simulink model "UrbanCHIL"  (Simulink 8.1)
settings: Solver=ode1  StartTime=0.0  StopTime=inf  FixedStep=Ts  MaxStep=1e-3  RelTol=1e-3
PostLoadFcn:
  | NREL_Mode=1; BANSHEE_init;
InitFcn:
  | NREL_Mode=1; BANSHEE_init;
values from neighbouring files (symbols this model uses):
  DER_REL = xlsread('DER_relay.xlsx')    [relay_settings_init.m]
  F0 = xlsread('F0_relay_banshee.xlsx')    [relay_settings_init.m]
  F2 = xlsread('F2_relay_banshee.xlsx')    [relay_settings_init.m]
  F3 = xlsread('F3_relay_banshee.xlsx')    [relay_settings_init.m]
  F4 = xlsread('F4_relay_nrel.xlsx')    [relay_settings_init.m]
  Ts = 100E-6    (= 0.0001)    [BANSHEE_init.m]    (also in Ghost_init.m)
undefined symbols (not defined in the file or in its folder): CBID, communications_lib, Feeder2_lib, Feeder3_lib, Feeder4_lib, generic_ethernet_cb, Left, relay_housing_lib, SM_UtilityService, SS_COMMUNICATION, SS_F2_RELAY_HOUSING, SS_F3_RELAY_HOUSING, SS_Feeder2, SS_Feeder3, SS_Feeder4, Stim, type, utility_service_lib, V
libraries: simulink x80, relay_modbus_lib x80, breaker_lib x46, rtio_generic_modbus x45, cables_lib x30, rtlab x22, Load_lib x21, powerlib x20, transformer_lib x19, ssn_lib x13, artemis x6, BESS_lib x4
(part 4 of 6)

== system UrbanCHIL/SC_ctrl/PV2 control ==
  note: Use Modbus from
      | Console
  note: Use Modbus TCP
  Bus Creator1 : BusCreator  Inputs=3
  Bus Creator12 : BusCreator  Inputs=8
  Gain3 : Gain  Gain=1000
  Gain4 : Gain  Gain=1000
  Gain5 : Gain  Gain=4800
  Gain6 : Gain  Gain=6000
  Manual Switch : ManualSwitch  CurrentSetting=0
  Manual Switch1 : ManualSwitch  CurrentSetting=0
  Manual Switch2 : ManualSwitch
  Manual Switch3 : ManualSwitch  CurrentSetting=0
  PCmd{1..2,4,6} (4 alike) : Constant  Value=0
  PCmd3 : Constant
  PCmd5 : Constant  Value=11
  PCmd7 : Constant
  PCmd8 : Constant
  Rate Transition : RateTransition  Deterministic=off
  S Profile1 : simulink/Sources/Repeating Sequence Stair  OutValues=Stim.PV2.Ena  tsamp=[Stim.Ts Ts]  OutMin=[]  OutMax=[]  OutDataTypeStr=Inherit: Inherit via back propagation  OutDataType=fixdt(0,8)  ConRadixGroup=Best Precision: Vector-wise  OutScaling=2^-12
  S Profile2 : simulink/Sources/Repeating Sequence Stair  OutValues=Stim.ESS2.p  tsamp=[Stim.Ts Ts]  OutMin=[]  OutMax=[]  OutDataTypeStr=Inherit: Inherit via back propagation  OutDataType=fixdt(0,8)  ConRadixGroup=Best Precision: Vector-wise  OutScaling=2^-12
  S Profile3 : simulink/Sources/Repeating Sequence Stair  OutValues=Stim.ESS2.q  tsamp=[Stim.Ts Ts]  OutMin=[]  OutMax=[]  OutDataTypeStr=Inherit: Inherit via back propagation  OutDataType=fixdt(0,8)  ConRadixGroup=Best Precision: Vector-wise  OutScaling=2^-12
  S Profile4 : simulink/Sources/Repeating Sequence Stair  OutValues=Stim.ESS2.v  tsamp=[Stim.Ts Ts]  OutMin=[]  OutMax=[]  OutDataTypeStr=Inherit: Inherit via back propagation  OutDataType=fixdt(0,8)  ConRadixGroup=Best Precision: Vector-wise  OutScaling=2^-12
  S Profile5 : simulink/Sources/Repeating Sequence Stair  OutValues=Stim.ESS2.f  tsamp=[Stim.Ts Ts]  OutMin=[]  OutMax=[]  OutDataTypeStr=Inherit: Inherit via back propagation  OutDataType=fixdt(0,8)  ConRadixGroup=Best Precision: Vector-wise  OutScaling=2^-12
  Tuning : Subsystem
  Out1 : Outport
  wires:
  Manual Switch3/1 -> Bus Creator12/1  "Ctrl"
  PCmd8/1 -> Manual Switch3/2
  S Profile5/1 -> Gain6/1
  Manual Switch/1 -> Gain3/1
  Bus Creator12/1 -> Bus Creator1/1  "ModbusFromSC"
  Manual Switch1/1 -> Gain4/1
  S Profile4/1 -> Gain5/1
  PCmd4/1 -> Manual Switch1/2
  PCmd3/1 -> Manual Switch/2
  S Profile2/1 -> Manual Switch/1
  S Profile3/1 -> Manual Switch1/1
  S Profile1/1 -> Manual Switch3/1
  PCmd1/1 -> Bus Creator12/6
  PCmd2/1 -> Bus Creator12/7
  PCmd5/1 -> Bus Creator12/8
  Bus Creator1/1 -> Rate Transition/1
  Manual Switch2/1 -> Bus Creator1/2  "ModbusEnable"
  PCmd6/1 -> Manual Switch2/1
  PCmd7/1 -> Manual Switch2/2
  Gain3/1 -> Bus Creator12/2  "PCmd"
  Gain4/1 -> Bus Creator12/3  "QCmd"
  Gain5/1 -> Bus Creator12/4  "VoltCmd"
  Gain6/1 -> Bus Creator12/5  "FreqCmd"
  Rate Transition/1 -> Out1/1
  Tuning/1(Tuning) -> Bus Creator1/3  "Tuning"

== system UrbanCHIL/SC_ctrl/Plots ==
  note: VRMSLL
      | Hz
      | kW
      | kVAR
  CMBNE_SGNLS : Inport
  Bus Selector1 : BusSelector  OutputSignals=F4_MS_IN.PV_DATA.pv_phil.Vdc,F4_MS_IN.PV_DATA.pv_phil.Idc,F4_MS_IN.PV_DATA.pv_phil.Pdc,F4_MS_IN.PV_DATA.pv_phil.Vref,F4_MS_IN.PV_DATA.pv_phil.Iref  OutputAsBus=on
  Bus Selector10 : BusSelector  OutputSignals=F2_MS_IN.PV_DATA.CB_meas.cb_meas.Status,F2_MS_IN.PV_DATA.CB_meas.relay_out.m.kw,F2_MS_IN.PV_DATA.CB_meas.relay_out.m.kvar,F2_MS_IN.PV_DATA.CB_meas.relay_out.m.Va_rms,F2_MS_IN.PV_DATA.CB_meas.relay_out.m.Hz  OutputAsBus=on
  Bus Selector11 : BusSelector  OutputSignals=F4_MS_IN.ESS_DATA.CB_meas.cb_meas.Status,F4_MS_IN.ESS_DATA.CB_meas.relay_out.m.kw,F4_MS_IN.ESS_DATA.CB_meas.relay_out.m.kvar,F4_MS_IN.ESS_DATA.CB_meas.relay_out.m.Va_rms,F4_MS_IN.ESS_DATA.CB_meas.relay_out.m.Hz,F4_MS_IN.ESS_DATA.Battery.SoC  OutputAsBus=on
  Bus Selector12 : BusSelector  OutputSignals=F4_MS_IN.PV_DATA.CB_meas.cb_meas.Status,F4_MS_IN.PV_DATA.CB_meas.relay_out.m.kw,F4_MS_IN.PV_DATA.CB_meas.relay_out.m.kvar,F4_MS_IN.PV_DATA.CB_meas.relay_out.m.Va_rms,F4_MS_IN.PV_DATA.CB_meas.relay_out.m.Hz  OutputAsBus=on
  Bus Selector13 : BusSelector  OutputSignals=F4_MS_IN.GEN3_DATA.cb.cb_meas.Status,F4_MS_IN.GEN3_DATA.cb.relay_out.m.kw,F4_MS_IN.GEN3_DATA.cb.relay_out.m.kvar,F4_MS_IN.GEN3_DATA.cb.relay_out.m.Va_rms,F4_MS_IN.GEN3_DATA.cb.relay_out.m.Hz  OutputAsBus=on
  Bus Selector2 : BusSelector  OutputSignals=F3_MS_IN.NG_CHP_DATA.cb.cb_meas.Status,F3_MS_IN.NG_CHP_DATA.cb.relay_out.m.kw,F3_MS_IN.NG_CHP_DATA.cb.relay_out.m.kvar,F3_MS_IN.NG_CHP_DATA.cb.relay_out.m.Va_rms,F3_MS_IN.NG_CHP_DATA.cb.relay_out.m.Hz  OutputAsBus=on
  Bus Selector4 : BusSelector  OutputSignals=F2_RELAY_OUT.F2_PCC
  Bus Selector6 : BusSelector  OutputSignals=m.Vpu,m.Hz,m.kw,m.kvar  OutputAsBus=on
  Bus Selector7 : BusSelector  OutputSignals=F3_RELAY_OUT.F3_PCC
  Bus Selector8 : BusSelector  OutputSignals=m.Vpu,m.Hz,m.kw,m.kvar  OutputAsBus=on
  Bus Selector9 : BusSelector  OutputSignals=F2_MS_IN.ESS_DATA.CB_meas.cb_meas.Status,F2_MS_IN.ESS_DATA.CB_meas.relay_out.m.kw,F2_MS_IN.ESS_DATA.CB_meas.relay_out.m.kvar,F2_MS_IN.ESS_DATA.CB_meas.relay_out.m.Va_rms,F2_MS_IN.ESS_DATA.CB_meas.relay_out.m.Hz,F2_MS_IN.ESS_DATA.Battery.SoC  OutputAsBus=on
  CHP : Display
  ESS : Display
  ESS2 : Display
  F2 : Display
  F3 : Display
  Gen3 : Display
  PV : Display
  PV2 : Display
  PV2_DC : Display
  wires:
  Bus Selector4/1 -> Bus Selector6/1  "<F2_PCC>"
  Bus Selector8/1 -> F3/1
  Bus Selector2/1 -> CHP/1
  CMBNE_SGNLS/1 -> [CMBNE_SGNLS]
  [CMBNE_SGNLS] -> Bus Selector4/1
  [CMBNE_SGNLS] -> Bus Selector7/1
  [CMBNE_SGNLS] -> Bus Selector2/1
  Bus Selector6/1 -> F2/1
  Bus Selector7/1 -> Bus Selector8/1  "<F3_PCC>"
  Bus Selector9/1 -> ESS/1
  [CMBNE_SGNLS] -> Bus Selector9/1
  Bus Selector10/1 -> PV/1
  [CMBNE_SGNLS] -> Bus Selector10/1
  Bus Selector11/1 -> ESS2/1
  [CMBNE_SGNLS] -> Bus Selector11/1
  Bus Selector12/1 -> PV2/1
  [CMBNE_SGNLS] -> Bus Selector12/1
  Bus Selector13/1 -> Gen3/1
  [CMBNE_SGNLS] -> Bus Selector13/1
  [CMBNE_SGNLS] -> Bus Selector1/1
  Bus Selector1/1 -> PV2_DC/1

== system UrbanCHIL/SC_ctrl/SOC1 control ==
  note: Use Modbus TCP
  note: Use Modbus from
      | Console
  SOC : Inport
  Bias : Bias  Bias=1
  Bus Creator1 : BusCreator  Inputs=3
  Bus Creator12 : BusCreator  Inputs=8
  Constant : Constant
  Constant1 : Constant
  Constant2 : Constant
  Constant3 : Constant  Value=50
  Gain : Gain  Gain=-0.01
  Gain1 : Gain  Gain=2
  Gain2 : Gain
  Gain5 : Gain  Gain=4800
  Gain6 : Gain  Gain=6000
  Manual Switch1 : ManualSwitch
  Manual Switch2 : ManualSwitch
  Manual Switch3 : ManualSwitch
  PCmd1 : Constant  Value=300
  PCmd2 : Constant  Value=300
  PCmd3 : Constant  Value=0
  PCmd4 : Constant  Value=0
  PCmd5 : Constant  Value=13
  PCmd6 : Constant  Value=0
  PCmd7 : Constant
  PCmd8 : Constant  Value=3
  PCmd9 : Constant  Value=1.003
  Rate Transition : RateTransition  Deterministic=off
  Rate Transition1 : RateTransition  Deterministic=off  OutPortSampleTime=100e-3
  Saturation : Saturate  UpperLimit=6045  LowerLimit=5955
  Sum : Sum  Inputs=++|
  Sum1 : Sum  Inputs=+-|
  Tuning : Subsystem
  Out1 : Outport
  wires:
  PCmd8/1 -> Manual Switch3/2
  Manual Switch3/1 -> Bus Creator12/1  "Ctrl"
  Gain6/1 -> Saturation/1
  Gain5/1 -> Bus Creator12/4  "VoltCmd"
  PCmd4/1 -> Bus Creator12/3  "QCmd"
  PCmd3/1 -> Bus Creator12/2  "PCmd"
  PCmd7/1 -> Manual Switch2/2
  PCmd6/1 -> Manual Switch2/1
  Manual Switch2/1 -> Bus Creator1/2  "ModbusEnable"
  Bus Creator1/1 -> Rate Transition/1
  PCmd5/1 -> Bus Creator12/8
  PCmd2/1 -> Bus Creator12/7
  PCmd1/1 -> Bus Creator12/6
  Sum/1 -> Manual Switch3/1
  Gain1/1 -> Sum/2
  Gain2/1 -> Sum/1
  Constant1/1 -> Gain5/1
  Constant2/1 -> Gain2/1  "Enable"
  Bus Creator12/1 -> Bus Creator1/1  "ModbusFromSC"
  Constant/1 -> Gain1/1  "GridBreaker"
  Rate Transition/1 -> Out1/1
  Saturation/1 -> Bus Creator12/5  "FreqCmd"
  Bias/1 -> Manual Switch1/1
  Constant3/1 -> Sum1/1
  SOC/1 -> Rate Transition1/1
  Sum1/1 -> Gain/1
  Gain/1 -> Bias/1
  Rate Transition1/1 -> Sum1/2
  Manual Switch1/1 -> Gain6/1
  PCmd9/1 -> Manual Switch1/2
  Tuning/1(Tuning) -> Bus Creator1/3  "Tuning"

== system UrbanCHIL/SC_ctrl/SOC2 control ==
  note: Use Modbus from
      | Console
  note: Use Modbus TCP
  SOC : Inport
  Bias : Bias  Bias=1
  Bus Creator1 : BusCreator  Inputs=3
  Bus Creator12 : BusCreator  Inputs=8
  Constant : Constant
  Constant1 : Constant
  Constant2 : Constant
  Constant3 : Constant  Value=50
  Gain : Gain  Gain=-0.01
  Gain1 : Gain  Gain=2
  Gain2 : Gain
  Gain5 : Gain  Gain=4800
  Gain6 : Gain  Gain=6000
  Manual Switch1 : ManualSwitch
  Manual Switch2 : ManualSwitch
  Manual Switch3 : ManualSwitch
  PCmd1 : Constant  Value=300
  PCmd2 : Constant  Value=300
  PCmd3 : Constant  Value=0
  PCmd4 : Constant  Value=0
  PCmd5 : Constant  Value=13
  PCmd6 : Constant  Value=0
  PCmd7 : Constant
  PCmd8 : Constant  Value=3
  PCmd9 : Constant  Value=1.003
  Rate Transition : RateTransition  Deterministic=off
  Rate Transition1 : RateTransition  Deterministic=off  OutPortSampleTime=100e-3
  Saturation : Saturate  UpperLimit=6045  LowerLimit=5955
  Sum : Sum  Inputs=++|
  Sum1 : Sum  Inputs=+-|
  Tuning : Subsystem
  Out1 : Outport
  wires:
  Sum1/1 -> Gain/1
  SOC/1 -> Rate Transition1/1
  Constant3/1 -> Sum1/1
  Bias/1 -> Manual Switch1/1
  Saturation/1 -> Bus Creator12/5  "FreqCmd"
  Rate Transition/1 -> Out1/1
  Constant/1 -> Gain1/1  "GridBreaker"
  Bus Creator12/1 -> Bus Creator1/1  "ModbusFromSC"
  Constant2/1 -> Gain2/1  "Enable"
  Constant1/1 -> Gain5/1
  Gain2/1 -> Sum/1
  Gain1/1 -> Sum/2
  Sum/1 -> Manual Switch3/1
  PCmd1/1 -> Bus Creator12/6
  PCmd2/1 -> Bus Creator12/7
  PCmd5/1 -> Bus Creator12/8
  Bus Creator1/1 -> Rate Transition/1
  Manual Switch2/1 -> Bus Creator1/2  "ModbusEnable"
  PCmd6/1 -> Manual Switch2/1
  PCmd7/1 -> Manual Switch2/2
  PCmd3/1 -> Bus Creator12/2  "PCmd"
  PCmd4/1 -> Bus Creator12/3  "QCmd"
  Gain5/1 -> Bus Creator12/4  "VoltCmd"
  Gain6/1 -> Saturation/1
  Manual Switch3/1 -> Bus Creator12/1  "Ctrl"
  PCmd8/1 -> Manual Switch3/2
  Gain/1 -> Bias/1
  Rate Transition1/1 -> Sum1/2
  Manual Switch1/1 -> Gain6/1
  PCmd9/1 -> Manual Switch1/2
  Tuning/1(Tuning) -> Bus Creator1/3  "Tuning"

== system UrbanCHIL/SC_ctrl/TestSeq ==
  TestData : Inport
  Bias : Bias  Bias=[0:-1:-10]*1.1
  Bias1 : Bias  Bias=[0:-1:-2]*1.1
  Bias2 : Bias  Bias=[0:-1:-1]*1.1
  Bias3 : Bias  Bias=[0:-1:-1]*1.1
  Bus Selector : BusSelector  OutputSignals=TestSeq.seq_time,TestSeq.fault,TestSeq.dms,TestSeq.grid,TestSeq.motor,TestSeq.misc
  Bus Selector1 : BusSelector  OutputSignals=loc1,loc2,loc3,loc4,loc5,loc6,gen1,gen2,gen3,pv1,pv2  OutputAsBus=on
  Bus Selector2 : BusSelector  OutputSignals=DisReq,kWEna,PFEna  OutputAsBus=on
  Bus Selector3 : BusSelector  OutputSignals=kWref,PFref
  Bus Selector4 : BusSelector  OutputSignals=Dp,Dq  OutputAsBus=on
  Bus Selector5 : BusSelector  OutputSignals=Hz,Volt  OutputAsBus=on
  Bus Selector6 : BusSelector  OutputSignals=ena1,ena2  OutputAsBus=on
  Bus Selector7 : BusSelector  OutputSignals=cut_grid,mgc_ena  OutputAsBus=on
  Bus Selector8 : BusSelector  OutputSignals=TestSeq.price,TestSeq.pv.insolation1,TestSeq.pv.insolation2  OutputAsBus=on
  Display : Display
  Gain : Gain  Gain=[1/60 1/115000]
  TestSequence : Scope  NumInputPorts=9
      settings: YMin=-5~-5~-5~-5~-5~-5~-5~-5~-5  YMax=5~5~5~5~5~5~5~5~5  Decimation=50
  ms2sek : Gain  Gain=0.001
  wires:
  Bus Selector8/1 -> TestSequence/9  "price, pv1, pv2"
  Bias3/1 -> TestSequence/8  "misc: cut_grid, mgc_ena"
  Bus Selector7/1 -> Bias3/1
  Bus Selector/6 -> Bus Selector7/1  "<misc>"
  Bias2/1 -> TestSequence/7  "motor: ena1, ena2"
  Bus Selector6/1 -> Bias2/1
  Bus Selector/5 -> Bus Selector6/1  "<motor>"
  Gain/1 -> TestSequence/6  "GridPU: Hz/Volt"
  Bus Selector5/1 -> Gain/1
  Bus Selector/4 -> Bus Selector5/1  "<grid>"
  Bus Selector/3 -> Bus Selector2/1, Bus Selector4/1, Bus Selector3/1  "<dms>"
  Bus Selector4/1 -> TestSequence/5  "Dp, Dq"
  Bus Selector3/2 -> TestSequence/4  "<PFref>"
  Bus Selector3/1 -> TestSequence/3  "<kWref>"
  Bias1/1 -> TestSequence/2  "dms: DisReq, kwCmd, PFCmd"
  Bus Selector2/1 -> Bias1/1
  Bias/1 -> TestSequence/1  "flt: loc1-6, gen1-3, ess1-2, pv1-2"
  Bus Selector1/1 -> Bias/1
  Bus Selector/2 -> Bus Selector1/1  "<fault>"
  Bus Selector/1 -> ms2sek/1  "<seq_time>"
  TestData/1 -> Bus Selector/1, Bus Selector8/1
  ms2sek/1 -> Display/1

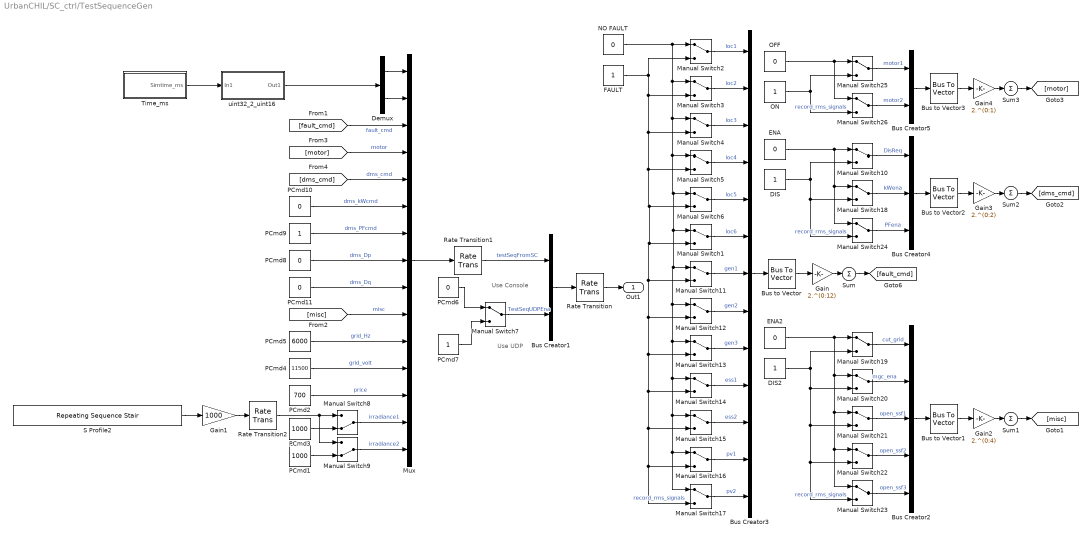
== system UrbanCHIL/SC_ctrl/TestSequenceGen ==
  note: Use UDP
  note: Use Console
  Bus Creator1 : BusCreator  Inputs=2
  Bus Creator2 : BusCreator  Inputs=5
  Bus Creator3 : BusCreator  Inputs=13
  Bus Creator4 : BusCreator  Inputs=3
  Bus Creator5 : BusCreator  Inputs=2
  Bus to Vector{,1..3} (4 alike) : BusToVector
  DIS : Constant
  DIS2 : Constant
  Demux : Demux  Outputs=2
  ENA : Constant  Value=0
  ENA2 : Constant  Value=0
  FAULT : Constant
  Gain : Gain  Gain=2.^(0:12)
  Gain1 : Gain  Gain=1000
  Gain2 : Gain  Gain=2.^(0:4)
  Gain3 : Gain  Gain=2.^(0:2)
  Gain4 : Gain  Gain=2.^(0:1)
  Manual Switch{1..7,10..26} (24 alike) : ManualSwitch
  Manual Switch8 : ManualSwitch  CurrentSetting=0
  Manual Switch9 : ManualSwitch  CurrentSetting=0
  Mux : Mux  Inputs=15
  NO FAULT : Constant  Value=0
  OFF : Constant  Value=0
  ON : Constant
  PCmd1 : Constant  Value=1000
  PCmd10 : Constant  Value=0
  PCmd11 : Constant  Value=0
  PCmd2 : Constant  Value=700
  PCmd3 : Constant  Value=1000
  PCmd4 : Constant  Value=11500
  PCmd5 : Constant  Value=6000
  PCmd6 : Constant  Value=0  SampleTime=[Stim.Ts Ts]
  PCmd7 : Constant
  PCmd8 : Constant  Value=0
  PCmd9 : Constant
  Rate Transition : RateTransition  Deterministic=off
  Rate Transition1 : RateTransition  Deterministic=off  OutPortSampleTime=10e-3
  Rate Transition2 : RateTransition  Deterministic=off  OutPortSampleTime=10e-3
  S Profile2 : simulink/Sources/Repeating Sequence Stair  OutValues=Stim.PV2.Irradiance  tsamp=[Stim.Ts Ts]  OutMin=[]  OutMax=[]  OutDataTypeStr=Inherit: Inherit via back propagation  OutDataType=fixdt(0,8)  ConRadixGroup=Best Precision: Vector-wise  OutScaling=2^-12
  Sum{,1..3} (4 alike) : Sum  Inputs=+
  Time_ms : Subsystem
  uint32_2_uint16 : Subsystem
      mask Display: disp('uint32_2_uint16');
  Out1 : Outport
  wires:
  Rate Transition1/1 -> Bus Creator1/1  "testSeqFromSC"
  uint32_2_uint16/1(Out1) -> Demux/1
  S Profile2/1 -> Gain1/1
  Sum3/1 -> [motor]
  Gain4/1 -> Sum3/1
  Bus to Vector3/1 -> Gain4/1
  OFF/1 -> Manual Switch26/1, Manual Switch25/1
  ON/1 -> Manual Switch25/2, Manual Switch26/2  "record_rms_signals"
  Manual Switch26/1 -> Bus Creator5/2  "motor2"
  Manual Switch25/1 -> Bus Creator5/1  "motor1"
  Bus Creator5/1 -> Bus to Vector3/1
  Sum2/1 -> [dms_cmd]
  Gain3/1 -> Sum2/1
  Bus to Vector2/1 -> Gain3/1
  ENA/1 -> Manual Switch10/1, Manual Switch18/1, Manual Switch24/1
  DIS/1 -> Manual Switch18/2, Manual Switch24/2, Manual Switch10/2  "record_rms_signals"
  Manual Switch18/1 -> Bus Creator4/2  "kWena"
  Manual Switch10/1 -> Bus Creator4/1  "DisReq"
  Bus Creator4/1 -> Bus to Vector2/1
  Manual Switch24/1 -> Bus Creator4/3  "PFena"
  Sum1/1 -> [misc]
  Gain2/1 -> Sum1/1
  Bus to Vector1/1 -> Gain2/1
  ENA2/1 -> Manual Switch23/1, Manual Switch22/1, Manual Switch21/1, Manual Switch20/1, Manual Switch19/1
  DIS2/1 -> Manual Switch19/2, Manual Switch23/2, Manual Switch22/2, Manual Switch21/2, Manual Switch20/2  "record_rms_signals"
  Manual Switch20/1 -> Bus Creator2/2  "mgc_ena"
  Manual Switch23/1 -> Bus Creator2/5  "open_ssf3"
  Manual Switch19/1 -> Bus Creator2/1  "cut_grid"
  Bus Creator2/1 -> Bus to Vector1/1
  Manual Switch22/1 -> Bus Creator2/4  "open_ssf2"
  Manual Switch21/1 -> Bus Creator2/3  "open_ssf1"
  PCmd11/1 -> Mux/9  "dms_Dq"
  PCmd10/1 -> Mux/6  "dms_kWcmd"
  PCmd9/1 -> Mux/7  "dms_PFcmd"
  PCmd8/1 -> Mux/8  "dms_Dp"
  [dms_cmd] -> Mux/5  "dms_cmd"
  [motor] -> Mux/4  "motor"
  [misc] -> Mux/10  "misc"
  PCmd5/1 -> Mux/11  "grid_Hz"
  PCmd4/1 -> Mux/12  "grid_volt"
  Demux/2 -> Mux/2
  Demux/1 -> Mux/1
  Time_ms/1(Simtime_ms) -> uint32_2_uint16/1(In1)
  Gain1/1 -> Rate Transition2/1
  PCmd2/1 -> Mux/13  "price"
  Manual Switch8/1 -> Mux/14  "irradiance1"
  PCmd1/1 -> Manual Switch9/2
  Manual Switch9/1 -> Mux/15  "irradiance2"
  PCmd3/1 -> Manual Switch8/2
  Rate Transition/1 -> Out1/1
  PCmd7/1 -> Manual Switch7/2
  PCmd6/1 -> Manual Switch7/1
  Manual Switch7/1 -> Bus Creator1/2  "TestSeqUDPEna"
  Bus Creator1/1 -> Rate Transition/1
  Mux/1 -> Rate Transition1/1
  Sum/1 -> [fault_cmd]
  Gain/1 -> Sum/1
  Bus to Vector/1 -> Gain/1
  Manual Switch17/1 -> Bus Creator3/13  "pv2"
  Manual Switch16/1 -> Bus Creator3/12  "pv1"
  NO FAULT/1 -> Manual Switch2/1, Manual Switch3/1, Manual Switch4/1, Manual Switch5/1, Manual Switch6/1, Manual Switch1/1, Manual Switch11/1, Manual Switch16/1, Manual Switch17/1, Manual Switch15/1, Manual Switch14/1, Manual Switch13/1, Manual Switch12/1
  FAULT/1 -> Manual Switch3/2, Manual Switch4/2, Manual Switch5/2, Manual Switch6/2, Manual Switch11/2, Manual Switch15/2, Manual Switch16/2, Manual Switch17/2, Manual Switch14/2, Manual Switch13/2, Manual Switch12/2, Manual Switch1/2, Manual Switch2/2  "record_rms_signals"
  Manual Switch12/1 -> Bus Creator3/8  "gen2"
  Manual Switch15/1 -> Bus Creator3/11  "ess2"
  Manual Switch11/1 -> Bus Creator3/7  "gen1"
  Manual Switch14/1 -> Bus Creator3/10  "ess1"
  Manual Switch13/1 -> Bus Creator3/9  "gen3"
  Manual Switch1/1 -> Bus Creator3/6  "loc6"
  Manual Switch3/1 -> Bus Creator3/2  "loc2"
  Manual Switch6/1 -> Bus Creator3/5  "loc5"
  Manual Switch2/1 -> Bus Creator3/1  "loc1"
  Bus Creator3/1 -> Bus to Vector/1
  [fault_cmd] -> Mux/3  "fault_cmd"
  Manual Switch5/1 -> Bus Creator3/4  "loc4"
  Manual Switch4/1 -> Bus Creator3/3  "loc3"
  Rate Transition2/1 -> Manual Switch8/1, Manual Switch9/1

== system UrbanCHIL/SS_COMMUNICATION/BESS_data ==
  note: 0 .... 10000
      | 0 ... 100%
  Bus Selector1 : BusSelector  OutputSignals=Battery.SoC
  Bus Selector2 : BusSelector  OutputSignals=Battery.SoC
  Bus Selector3 : BusSelector  OutputSignals=ESS_DATA
  Bus Selector9 : BusSelector  OutputSignals=ESS_DATA
  Mux : Mux  Inputs=2
  Scale_SoC : Gain  Gain=100
  Out1 : Outport
  wires:
  Mux/1 -> Scale_SoC/1
  Bus Selector1/1 -> Mux/2  "<SoC>"
  Bus Selector9/1 -> Bus Selector1/1  "<ESS_DATA>"
  [F4_MS_IN] -> Bus Selector9/1
  Scale_SoC/1 -> Out1/1
  Bus Selector2/1 -> Mux/1  "<SoC>"
  Bus Selector3/1 -> Bus Selector2/1  "<ESS_DATA>"
  [F2_MS_IN] -> Bus Selector3/1

== system UrbanCHIL/SS_COMMUNICATION/DieselData ==
  Bus Selector : BusSelector  OutputSignals=GEN3_DATA.gen.gal_per_hr,GEN3_DATA.cb.relay_out.m.Vpu
  Constant : Constant  Value=0
  Constant1 : Constant  Value=0
  Mux : Mux
  scale_diesel3 : Gain  Gain=100
  Out2 : Outport
  wires:
  Bus Selector/2 -> Mux/4  "<Vpu>"
  Mux/1 -> scale_diesel3/1
  Constant/1 -> Mux/1
  Bus Selector/1 -> Mux/2  "<gal_per_hr>"
  [F4_MS_IN] -> Bus Selector/1
  scale_diesel3/1 -> Out2/1
  Constant1/1 -> Mux/3

== system UrbanCHIL/SS_COMMUNICATION/GOOSE_RX  ==
  Bus Creator2 : BusCreator  Inputs=3
  Bus Creator3 : BusCreator  Inputs=7
  Bus Creator4 : BusCreator  Inputs=8
  Bus Creator5 : BusCreator  Inputs=9
  Bus Creator7 : BusCreator
  Bus Creator8 : BusCreator  Inputs=5
  Constant{1..29,32..33} (31 alike) : Constant  Value=0
  MGC_Message : Outport
  wires:
  Constant18/1 -> Bus Creator3/1  "Status"
  Bus Creator3/1 -> MGC_Message/1
  Constant1/1 -> Bus Creator2/1  "CB100"
  Constant3/1 -> Bus Creator2/2  "CB200"
  Constant2/1 -> Bus Creator2/3  "CB300"
  Bus Creator2/1 -> Bus Creator3/2  "PCC"
  Constant7/1 -> Bus Creator4/3  "CB108"
  Constant6/1 -> Bus Creator4/4  "CB109"
  Constant4/1 -> Bus Creator4/2  "CB107"
  Constant9/1 -> Bus Creator4/5  "CB110"
  Constant5/1 -> Bus Creator4/1  "CB104"
  Constant8/1 -> Bus Creator4/6  "CB111"
  Constant11/1 -> Bus Creator4/7  "CB113"
  Constant10/1 -> Bus Creator4/8  "CB114"
  Bus Creator4/1 -> Bus Creator3/3  "F1"
  Constant21/1 -> Bus Creator5/9  "CB219"
  Constant24/1 -> Bus Creator5/6  "CB216"
  Constant17/1 -> Bus Creator5/7  "CB217"
  Constant25/1 -> Bus Creator5/5  "CB213"
  Constant16/1 -> Bus Creator5/8  "CB218"
  Constant15/1 -> Bus Creator5/3  "CB208"
  Constant13/1 -> Bus Creator5/1  "CB204"
  Constant14/1 -> Bus Creator5/4  "CB212"
  Constant12/1 -> Bus Creator5/2  "CB206"
  Bus Creator5/1 -> Bus Creator3/4  "F2"
  Bus Creator8/1 -> Bus Creator3/6  "F4"
  Constant28/1 -> Bus Creator8/5  "CB406"
  Constant26/1 -> Bus Creator8/3  "CB403"
  Bus Creator7/1 -> Bus Creator3/5  "F3"
  Constant33/1 -> Bus Creator7/4  "CB310"
  Constant22/1 -> Bus Creator7/3  "CB309"
  Constant23/1 -> Bus Creator7/2  "CB308"
  Constant20/1 -> Bus Creator7/1  "CB307"
  Constant19/1 -> Bus Creator3/7  "NA"
  Constant29/1 -> Bus Creator8/4  "CB405"
  Constant27/1 -> Bus Creator8/2  "CB402"
  Constant32/1 -> Bus Creator8/1  "CB401"

== system UrbanCHIL/SS_COMMUNICATION/MGC_controller ==
  Bus Selector : BusSelector  OutputSignals=F4_CB_CTRL
  Bus Selector1 : BusSelector  OutputSignals=GEN3_DATA,ESS_DATA,PV_DATA
  Bus Selector{3..4,10..11} (4 alike) : BusSelector  OutputSignals=raw
  Bus Selector12 : BusSelector  OutputSignals=F3_CB_CTRL
  Bus Selector13 : BusSelector  OutputSignals=signal1,signal2,signal3,signal4,signal5,signal6,signal7,signal8,signal9,signal10  OutputAsBus=on
  Bus Selector14 : BusSelector  OutputSignals=F2_CB_CTRL
  Bus Selector15 : BusSelector  OutputSignals=signal1,signal2,signal3,signal4,signal5,signal6,signal7,signal8,signal9,signal10,signal11,signal12,signal13,signal14,signal15,signal16,signal17,signal18,signal19  OutputAsBus=on
  Bus Selector2 : BusSelector  OutputSignals=ctrl.raw
  Bus Selector7 : BusSelector  OutputSignals=ctrl.raw
  Bus Selector8 : BusSelector  OutputSignals=NG_CHP_DATA
  Bus Selector9 : BusSelector  OutputSignals=ESS_DATA,PV_DATA
  Bus to Vector : BusToVector
  Bus to Vector1 : BusToVector
  Bus to Vector2 : BusToVector
  Constant : Constant  Value=zeros(1,14)
  Constant4 : Constant  Value=zeros(1,8)
  Subsystem : Subsystem
      mask Display: disp('PCC control');
  Vector Concatenate : Concatenate  NumInputs=12
  MGC_controller : Outport
  wires:
  Bus Selector2/1 -> Vector Concatenate/10  "<raw>"
  Bus Selector3/1 -> Vector Concatenate/11  "<raw>"
  Bus Selector1/3 -> Bus Selector4/1  "<PV_DATA>"
  Bus Selector1/2 -> Bus Selector3/1  "<ESS_DATA>"
  Bus Selector1/1 -> Bus Selector2/1  "<GEN3_DATA>"
  [F4_MS_IN] -> Bus Selector1/1
  [F4_RELAY_OUT] -> Bus Selector/1
  Bus Selector/1 -> Bus to Vector/1  "<F4_CB_CTRL>"
  Bus to Vector1/1 -> Vector Concatenate/3
  Subsystem/1(Out1) -> Vector Concatenate/5
  Vector Concatenate/1 -> MGC_controller/1
  Bus Selector7/1 -> Vector Concatenate/9  "<raw>"
  [F3_MS_IN] -> Bus Selector8/1
  Bus Selector8/1 -> Bus Selector7/1  "<NG_CHP_DATA>"
  Bus Selector4/1 -> Vector Concatenate/12  "<raw>"
  [F2_MS_IN] -> Bus Selector9/1
  Bus Selector10/1 -> Vector Concatenate/7  "<raw>"
  Bus Selector11/1 -> Vector Concatenate/8  "<raw>"
  Bus Selector9/1 -> Bus Selector10/1  "<ESS_DATA>"
  Bus Selector9/2 -> Bus Selector11/1  "<PV_DATA>"
  Bus to Vector/1 -> Vector Concatenate/4
  [F3_RELAY_OUT] -> Bus Selector12/1
  Bus Selector12/1 -> Bus Selector13/1  "<F3_CB_CTRL>"
  Bus Selector13/1 -> Bus to Vector1/1
  Bus to Vector2/1 -> Vector Concatenate/2
  [F2_RELAY_OUT] -> Bus Selector14/1
  Bus Selector14/1 -> Bus Selector15/1  "<F2_CB_CTRL>"
  Bus Selector15/1 -> Bus to Vector2/1
  Constant/1 -> Vector Concatenate/1
  Constant4/1 -> Vector Concatenate/6

== system UrbanCHIL/SS_COMMUNICATION/Misc_data ==
  note: Data ordered as:
      | I-P-C
      | kW-VRMSLL
  Bus Creator : BusCreator
  Constant : Constant  Value=zeros(1,9)
  Constant1 : Constant  Value=0
  Mux8 : Mux  Inputs=2
  Mux9 : Mux  Inputs=2
  Subsystem : Subsystem
  Subsystem1 : Subsystem
  scale_load : Gain
  Out1 : Outport
  wires:
  scale_load/1 -> Mux9/1
  [F3_MS_IN] -> Bus Creator/2  "F3"
  [F2_MS_IN] -> Bus Creator/3  "F2"
  Constant1/1 -> Bus Creator/4  "F1"
  Bus Creator/1 -> Subsystem1/1(In1), Subsystem/1(In1)
  Mux8/1 -> scale_load/1
  Constant/1 -> Mux9/2
  Mux9/1 -> Out1/1
  [F4_MS_IN] -> Bus Creator/1  "F4"
  Subsystem/1(Out1) -> Mux8/1
  Subsystem1/1(Out1) -> Mux8/2

== system UrbanCHIL/SS_COMMUNICATION/Motor_data ==
  note: kW
      | kVAR
      | VLL_RMS
      | RPM
  Bus Selector3 : BusSelector  OutputSignals=MOTOR_DATA
  Bus Selector4 : BusSelector  OutputSignals=kW,kVAr,VRMSLL,RPM  OutputAsBus=on
  Bus to Vector1 : BusToVector
  Constant : Constant  Value=zeros(4,1)
  Mux5 : Mux  Inputs=2
  motor_data : Outport
  wires:
  Mux5/1 -> motor_data/1
  Constant/1 -> Mux5/1  "Motor1"
  Bus to Vector1/1 -> Mux5/2  "Motor2"
  [F3_MS_IN] -> Bus Selector3/1
  Bus Selector3/1 -> Bus Selector4/1  "<MOTOR_DATA>"
  Bus Selector4/1 -> Bus to Vector1/1

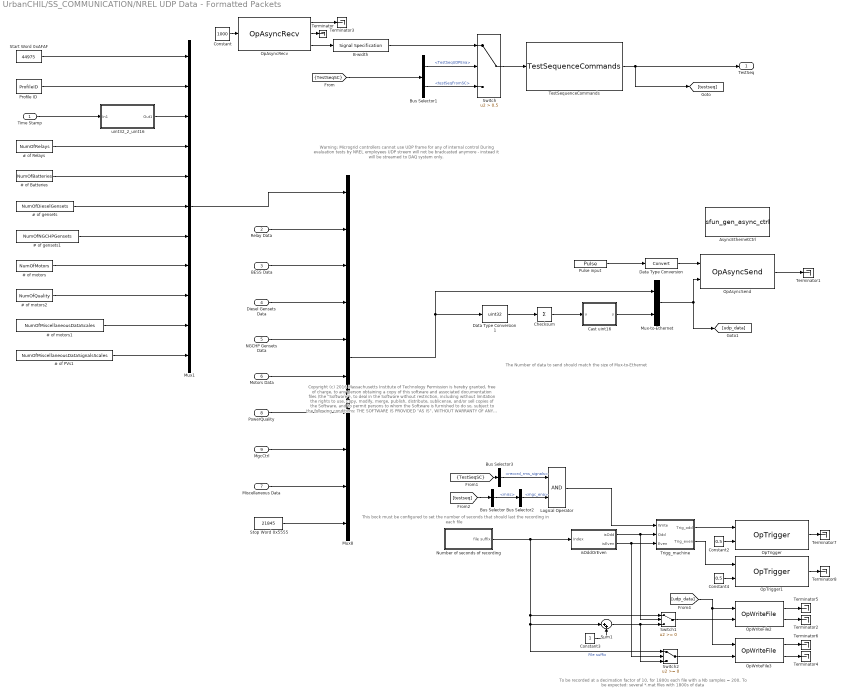
== system UrbanCHIL/SS_COMMUNICATION/NREL UDP Data - Formatted Packets ==
  note: The Number of data to send should match the size of Mux-to-Ethernet
  note: Copyright (c) 2016 Massachusetts Institute of Technology
      | Permission is hereby granted, free of charge, to any person obtaining a copy of this software and associated documentation files (the "Software"), to deal
      | in the Software without restriction, including without limitation the rights to use, copy, modify, merge, publish, distribute, sublicense, and/or sell copies of the
      | Software, and to permit persons to whom the Software is furnished to do so, subject to the following conditions:
      |
      | THE SOFTWARE IS PROVIDED "AS IS", WITHOUT WARRANTY OF ANY KIND, EXPRESS OR IMPLIED, INCLUDING BUT NOT LIMITED TO THE
      | WARRANTIES OF MERCHANTABILITY, FITNESS FOR A PARTICULAR PURPOSE AND NONINFRINGEMENT. IN NO EVENT SHALL THE AUTHORS
      | OR COPYRIGHT HOLDERS BE LIABLE FOR ANY CLAIM, DAMAGES OR OTHER LIABILITY, WHETHER IN AN ACTION OF CONTRACT, TORT OR
      | OTHERWISE, ARISING FROM, OUT OF OR IN CONNECTION WITH THE SOFTWARE OR THE USE OR OTHER DEALINGS IN THE SOFTWARE
  note: Warning: Microgrid controllers cannot use UDP frame for any of internal control
      | During evaluation tests by NREL employees UDP streem will not be bradcasted anymore - instead it will
      | be streamed to DAQ system only.
  note: This bock must be configured to set the number of
      | seconds that should last the recording in each file
  note: To be recorded at a decimation factor of 10,   for 1800s each file with a Nb samples = 200.
      | To be expected: several *.mat files with 1800s of data
  Time Stamp : Inport
  Relay Data : Inport  Port=2
  BESS Data : Inport  Port=3
  Diesel Gensets Data : Inport  Port=4
  NGCHP Gensets Data : Inport  Port=5
  Motors Data : Inport  Port=6
  Miscellaneous Data : Inport  Port=7
  "PowerQuality " : Inport  Port=8
  MgcCtrl : Inport  Port=9
  " # of motors" : Constant  Value=NumOfMotors  OutDataTypeStr=double
  " # of motors1" : Constant  Value=NumOfMiscellaneousDataScales  OutDataTypeStr=double
  " # of motors2" : Constant  Value=NumOfQuality  OutDataTypeStr=double
  # of Batteries : Constant  Value=NumOfBatteries  OutDataTypeStr=double
  # of PVs1 : Constant  Value=NumOfMiscellaneousDataSignalsScales  OutDataTypeStr=double
  # of Relays : Constant  Value=NumOfRelays  OutDataTypeStr=double
  # of gensets : Constant  Value=NumOfDieselGensets  OutDataTypeStr=double
  # of gensets1 : Constant  Value=NumOfNGCHPGensets  OutDataTypeStr=double
  AsyncEthernetCtrl : S-Function  InitFcn=generic_ethernet_cb('initfcn');  FunctionName=sfun_gen_async_ctrl  Parameters=ctrl_id, nbr_to_remote_endpoint, type_to_remote_endpoint,nbr_from_remote_endpoint,type_from_remote_endpoint,protocol,tcp_mode, port, offset_to_remote_endpoint,offset_from_remote_endpoint,swap_tx,swap_rx,0,nic_name,remote_ip,'','','','','','','','','','',exe_name,0  EnableBusSupport=off  mask(AsyncEthernetCtrl){ctrl_id=1, nbr_to_remote_endpoint=565, type_to_remote_endpoint=INT16, offset_to_remote_endpoint=0, nbr_from_remote_endpoint=15, type_from_remote_endpoint=INT16, offset_from_remote_endpoint=0, nic_name=eth1, protocol=UDP, tcp_mode=Server, port=7200, remote_ip=255.255.255.255, exe_name=AsyncEthernet, swap_tx=on, swap_rx=on}
      mask prompts: ctrl_id "Controller ID"; nbr_to_remote_endpoint "Number of data to send"; type_to_remote_endpoint "Type of data to send"; offset_to_remote_endpoint "Byte offset of transmission buffer"; nbr_from_remote_endpoint "Number of data expected to be received"; type_from_remote_endpoint "Type of data expected to be received"; offset_from_remote_endpoint "Byte offset of reception buffer"; nic_name "Network interface name"; tcp_mode "TCP mode"; remote_ip "Remote IP address"; exe_name "Name of the executable"; swap_tx "Swap data endianness before transmission"; swap_rx "Swap data endianness after reception"
      mask help: Generic asynchronous process configuration block
      mask Help: eval('rtlab_help(''opasyncgenctrl'');');
      mask TypeOptions type_to_remote_endpoint: UINT8 | INT8 | UINT16 | INT16 | UINT32 | INT32 | FLOAT | DOUBLE
      mask TypeOptions type_from_remote_endpoint: UINT8 | INT8 | UINT16 | INT16 | UINT32 | INT32 | FLOAT | DOUBLE
      mask TypeOptions protocol: UDP | TCP
      mask TypeOptions tcp_mode: Client | Server
      mask Display: disp(sprintf('\nEthernet communication \ninterface controller\n'))
  B-width : SignalSpecification  Dimensions=15
  Bus Selector : BusSelector  OutputSignals=misc
  Bus Selector1 : BusSelector  OutputSignals=TestSeq.TestSeqUDPEna,TestSeq.testSeqFromSC
  Bus Selector2 : BusSelector  OutputSignals=mgc_ena
  Bus Selector3 : BusSelector  OutputSignals=DataLogging.record_rms_signals
  Cast uint16 : MATLAB Function  TreatAsAtomicUnit=on
  Checksum : Sum  Inputs=+
  Constant : Constant  Value=1000
  Constant2 : Constant  Value=0.5
  Constant3 : Constant
  Constant4 : Constant  Value=0.5
  Data Type Conversion : DataTypeConversion
  Data Type Conversion1 : DataTypeConversion  OutDataTypeStr=uint32  ConvertRealWorld=Stored Integer (SI)  RndMeth=Nearest
  Logical Operator : Logic  AllPortsSameDT=off  OutDataTypeStr=boolean
  Mux-to-Ethernet : Mux  Inputs=2
  Mux1 : Mux  Inputs=11
  Mux8 : Mux  Inputs=10
  Number of seconds of recording : Subsystem  mask{time_s=60}
      mask prompts: time_s "Time in seconds"
      mask help: Set the number of seconds that should last the recording in each file.
  OpAsyncRecv : rtlab/Communication/Asynchronous/OpAsyncRecv  ctl_id=1  recv_id=1  enable_param=off  fp1=1  fp2=2  fp3=3  fp4=4  fp5=5  sp1=string1  sp2=string2  sp3=string3  sp4=string4  sp5=string5
  OpAsyncSend : rtlab/Communication/Asynchronous/OpAsyncSend  ctl_id=1  send_id=1  mode=DONT_NEED_REPLY  enable_param=off  fp1=1  fp2=2  fp3=3  fp4=4  fp5=5  sp1=string1  sp2=string2  sp3=string3  sp4=string4  sp5=string5
  OpTrigger : rtlab/DataLogging/OpTrigger  Trig_Type=TRIGGER SIGNAL >= TRIGGER LEVEL  Trig_Offset=0  Acq_Group=28
  OpTrigger1 : rtlab/DataLogging/OpTrigger  Trig_Type=TRIGGER SIGNAL >= TRIGGER LEVEL  Trig_Offset=0  Acq_Group=29
  OpWriteFile2 : rtlab/DataLogging/OpWriteFile  Static_File=off  varname=recVar  Filename=A_FILE_RECORDED_o.mat  rtpath='./'  nrtpath='.\'  Acq_Group=28  file_size=1000000000  write_offline=off  Sim_Mode=off  Nb_Samples=30500  Buffer_size=0
      settings: Decimation=20
  OpWriteFile3 : rtlab/DataLogging/OpWriteFile  Static_File=off  varname=recVar  Filename=A_FILE_RECORDED_e.mat  rtpath='./'  nrtpath='.\'  Acq_Group=29  file_size=1000000000  write_offline=off  Sim_Mode=off  Nb_Samples=30500  Buffer_size=0
      settings: Decimation=20
  Profile ID : Constant  Value=ProfileID  OutDataTypeStr=double
  Pulse input : DiscretePulseGenerator  PulseType=Time based  Period=1/5  PulseWidth=1/20
  Start Word 0xAFAF : Constant  Value=44975  OutDataTypeStr=double
  Stop Word 0x5555 : Constant  Value=21845  OutDataTypeStr=double
  Sum1 : Sum  Inputs=|++
  Switch : Switch  Criteria=u2 > Threshold  Threshold=0.5
  Switch1 : Switch
  Switch2 : Switch
  Terminator{,1..8} (9 alike) : Terminator
  TestSequenceCommands : TestSeq_slave_lib/TestSequenceCommands
  Trigg_machine : Subsystem
  isOddOrEven : Subsystem
  uint32_2_uint16 : Subsystem
      mask Display: disp('uint32_2_uint16');
  TestSeq : Outport
  wires:
  Start Word 0xAFAF/1 -> Mux1/1
  Pulse input/1 -> Data Type Conversion/1
  Mux1/1 -> Mux8/1
  Checksum/1 -> Cast uint16/1(u)
  Cast uint16/1(y) -> Mux-to-Ethernet/2
  Data Type Conversion1/1 -> Checksum/1
  BESS Data/1 -> Mux8/3
  Diesel Gensets Data/1 -> Mux8/4
  Relay Data/1 -> Mux8/2
  Mux8/1 -> Mux-to-Ethernet/1, Data Type Conversion1/1
  Stop Word 0x5555/1 -> Mux8/10
  NGCHP Gensets Data/1 -> Mux8/5
  Miscellaneous Data/1 -> Mux8/9
  Motors Data/1 -> Mux8/6
  Time Stamp/1 -> uint32_2_uint16/1(In1)
  # of PVs1/1 -> Mux1/11
  " # of motors1"/1 -> Mux1/10
  # of gensets1/1 -> Mux1/7
  # of gensets/1 -> Mux1/6
  " # of motors"/1 -> Mux1/8
  # of Batteries/1 -> Mux1/5
  # of Relays/1 -> Mux1/4
  Profile ID/1 -> Mux1/2
  Mux-to-Ethernet/1 -> [udp_data], OpAsyncSend/2
  Data Type Conversion/1 -> OpAsyncSend/1
  OpAsyncSend/1 -> Terminator1/1
  OpAsyncRecv/1 -> Terminator3/1
  Constant/1 -> OpAsyncRecv/1
  OpAsyncRecv/2 -> Terminator/1
  OpAsyncRecv/3 -> B-width/1
  B-width/1 -> Switch/1
  TestSequenceCommands/1 -> [testseq], TestSeq/1
  uint32_2_uint16/1(Out1) -> Mux1/3
  [TestSeqSC] -> Bus Selector1/1
  Bus Selector1/2 -> Switch/3  "<testSeqFromSC>"
  Bus Selector1/1 -> Switch/2  "<TestSeqUDPEna>"
  Switch/1 -> TestSequenceCommands/1
  " # of motors2"/1 -> Mux1/9
  "PowerQuality "/1 -> Mux8/7
  MgcCtrl/1 -> Mux8/8
  Bus Selector/1 -> Bus Selector2/1  "<misc>"
  Bus Selector2/1 -> Logical Operator/2  "<mgc_ena>"
  [TestSeqSC] -> Bus Selector3/1
  Bus Selector3/1 -> Logical Operator/1  "<record_rms_signals>"
  [udp_data] -> OpWriteFile2/1, OpWriteFile3/1
  Trigg_machine/1(Trig_odd) -> OpTrigger/1
  Trigg_machine/2(Trig_even) -> OpTrigger1/1
  Constant2/1 -> OpTrigger/2
  Constant4/1 -> OpTrigger1/2
  isOddOrEven/1(isOdd) -> Switch1/2, Trigg_machine/2(Odd)
  isOddOrEven/2(isEven) -> Switch2/2, Trigg_machine/3(Even)
  Switch1/1 -> OpWriteFile2/2
  Switch2/1 -> OpWriteFile3/2
  Constant3/1 -> Sum1/2
  Sum1/1 -> Switch1/3, Switch2/3
  Number of seconds of recording/1(file suffix) -> isOddOrEven/1(Index), Sum1/1, Switch2/1, Switch1/1  "File suffix"
  Logical Operator/1 -> Trigg_machine/1(Write)
  OpWriteFile2/2 -> Terminator2/1
  OpWriteFile3/2 -> Terminator4/1
  [testseq] -> Bus Selector/1
  OpWriteFile2/1 -> Terminator5/1
  OpWriteFile3/1 -> Terminator6/1
  OpTrigger1/1 -> Terminator8/1
  OpTrigger/1 -> Terminator7/1

== system UrbanCHIL/SS_COMMUNICATION/Power_quality_data ==
  Rst : Inport
  Bus Selector1 : BusSelector  OutputSignals=F3_CB_1.m.Hz,F3_CB_5.m.Hz,F3_CB_7.m.Hz,F3_CB_8.m.Hz,F3_CB_9.m.Hz  OutputAsBus=on
  Bus Selector2 : BusSelector  OutputSignals=F4_CB_1.m.Vpu,F4_CB_2.m.Vpu,F4_CB_5.m.Vpu  OutputAsBus=on
  Bus Selector3 : BusSelector  OutputSignals=F2_CB_1.m.Hz,F2_CB_6.m.Hz,F2_CB_8.m.Hz,F2_CB_9.m.Hz,F2_CB_12.m.Hz,F2_CB_14.m.Hz,F2_CB_16.m.Hz,F2_CB_17.m.Hz,F2_CB_19.m.Hz  OutputAsBus=on
  Bus Selector5 : BusSelector  OutputSignals=F3_CB_1.m.Vpu,F3_CB_5.m.Vpu,F3_CB_7.m.Vpu,F3_CB_8.m.Vpu,F3_CB_9.m.Vpu  OutputAsBus=on
  Bus Selector6 : BusSelector  OutputSignals=F2_CB_1.m.Vpu,F2_CB_6.m.Vpu,F2_CB_8.m.Vpu,F2_CB_9.m.Vpu,F2_CB_12.m.Vpu,F2_CB_14.m.Vpu,F2_CB_16.m.Vpu,F2_CB_17.m.Vpu,F2_CB_19.m.Vpu  OutputAsBus=on
  Bus Selector7 : BusSelector  OutputSignals=F4_CB_1.m.Hz,F4_CB_2.m.Hz,F4_CB_5.m.Hz  OutputAsBus=on
  Bus to Vector{,1..3,5..6} (6 alike) : BusToVector
  Constant3 : Constant  Value=zeros(1,6)
  IEEE1547a_Hz : power_quality_lib/IEEE1547a_Hz
  IEEE1547a_Volt : power_quality_lib/IEEE1547a_Volt
  Mux1 : Mux
  Mux2 : Mux
  Mux3 : Mux  Inputs=2
  Out1 : Outport
  wires:
  Rst/1 -> IEEE1547a_Volt/2, IEEE1547a_Hz/2
  Bus Selector7/1 -> Bus to Vector/1
  Mux3/1 -> Out1/1
  IEEE1547a_Volt/1 -> Mux3/2
  IEEE1547a_Hz/1 -> Mux3/1
  Bus to Vector/1 -> Mux1/4
  [F4_RELAY_OUT] -> Bus Selector2/1
  [F4_RELAY_OUT] -> Bus Selector7/1
  Bus Selector2/1 -> Bus to Vector3/1
  Bus to Vector3/1 -> Mux2/4
  [F2_RELAY_OUT] -> Bus Selector3/1
  [F3_RELAY_OUT] -> Bus Selector1/1
  Bus Selector3/1 -> Bus to Vector2/1
  Bus Selector1/1 -> Bus to Vector1/1
  Bus to Vector2/1 -> Mux1/2
  Bus to Vector1/1 -> Mux1/3
  Mux1/1 -> IEEE1547a_Hz/1
  [F3_RELAY_OUT] -> Bus Selector5/1
  Bus Selector5/1 -> Bus to Vector5/1
  Bus to Vector5/1 -> Mux2/3
  [F2_RELAY_OUT] -> Bus Selector6/1
  Bus Selector6/1 -> Bus to Vector6/1
  Bus to Vector6/1 -> Mux2/2
  Constant3/1 -> Mux2/1, Mux1/1
  Mux2/1 -> IEEE1547a_Volt/1

== system UrbanCHIL/SS_COMMUNICATION/Relay_data ==
  Constant : Constant  Value=zeros(1,14*5)
  ExtractF2 : Subsystem
      mask Display: disp('Generic F2 relays\nID = 15 .. 33')
  ExtractF3 : Subsystem
      mask Display: disp('Generic F3 relays\nID = 34 .. 43')
  ExtractF4 : Subsystem
      mask Display: disp('Generic F4 relays\nID = 44 .. 49')
  Mux12 : Mux  Inputs=5
  Scale_freq2 : Gain  Gain=100
  Sel_freq : Selector  InputPortWidth=59*5  IndexOptions=Index vector (dialog)  Indices=[4:5:59*5]  OutputSizes=1
  Sel_kvar : Selector  InputPortWidth=59*5  IndexOptions=Index vector (dialog)  Indices=[2:5:59*5]  OutputSizes=1
  Sel_kw : Selector  InputPortWidth=59*5  IndexOptions=Index vector (dialog)  Indices=[1:5:59*5]  OutputSizes=1
  Sel_status : Selector  InputPortWidth=59*5  IndexOptions=Index vector (dialog)  Indices=[5:5:59*5]  OutputSizes=1
  Sel_vpu : Selector  InputPortWidth=59*5  IndexOptions=Index vector (dialog)  Indices=[3:5:59*5]  OutputSizes=1
  Subsystem : Subsystem
      mask Display: disp('Generic PCC relays\nID = 50 .. 52')
  Subsystem1 : Subsystem
      mask Display: disp('GEN1,ESS1,PV1\nGEN2,GEN3,ESS2,PV1\nID = 53 .. 59')
  Vector Concatenate : Concatenate  NumInputs=6
  scale_kvar2 : Gain
  scale_kw2 : Gain
  scale_vpu2 : Gain  Gain=1000
  Out1 : Outport
  wires:
  [F3_RELAY_OUT] -> Subsystem/2(F3), ExtractF3/1(In1)
  [F2_RELAY_OUT] -> Subsystem/1(F2), ExtractF2/1(In1)
  [F4_RELAY_OUT] -> ExtractF4/1(In1)
  ExtractF4/1(Out1) -> Vector Concatenate/4
  ExtractF3/1(Out1) -> Vector Concatenate/3
  ExtractF2/1(Out1) -> Vector Concatenate/2
  Constant/1 -> Vector Concatenate/1
  Subsystem/1(Out1) -> Vector Concatenate/5
  [F4_MS_IN] -> Subsystem1/3(F4)
  [F3_MS_IN] -> Subsystem1/2(F3)
  [F2_MS_IN] -> Subsystem1/1(F2)
  Subsystem1/1(Out1) -> Vector Concatenate/6
  Mux12/1 -> Out1/1
  scale_kw2/1 -> Mux12/1
  scale_kvar2/1 -> Mux12/2
  Scale_freq2/1 -> Mux12/4
  scale_vpu2/1 -> Mux12/3
  Sel_kw/1 -> scale_kw2/1
  Sel_status/1 -> Mux12/5
  Sel_freq/1 -> Scale_freq2/1
  Sel_vpu/1 -> scale_vpu2/1
  Sel_kvar/1 -> scale_kvar2/1
  Vector Concatenate/1 -> Sel_status/1, Sel_freq/1, Sel_vpu/1, Sel_kvar/1, Sel_kw/1

== system UrbanCHIL/SS_COMMUNICATION/Time_ms ==
  Constant4 : Constant  Value=Ts/1e-3
  Sum : Sum  Inputs=++|
  Unit Delay : UnitDelay  SampleTime=-1
  Simtime_ms : Outport
  wires:
  Unit Delay/1 -> Sum/1
  Constant4/1 -> Sum/2
  Sum/1 -> Unit Delay/1, Simtime_ms/1

== system UrbanCHIL/SS_F2_RELAY_HOUSING/Subsystem ==
  bus : Inport
  Bus Selector35 : BusSelector  OutputSignals=NA,NA,NA,F2.CB204,NA,F2.CB206,NA,F2.CB208,NA,NA,NA,F2.CB212,F2.CB213,NA,NA,F2.CB216,F2.CB217,F2.CB218,F2.CB219,PCC.CB200
  Mux : Mux  Inputs=20
  vect : Outport
  wires:
  bus/1 -> Bus Selector35/1
  Mux/1 -> vect/1
  Bus Selector35/12 -> Mux/12  "<CB212>"
  Bus Selector35/17 -> Mux/17  "<CB217>"
  Bus Selector35/14 -> Mux/14  "<NA>"
  Bus Selector35/20 -> Mux/20  "<CB200>"
  Bus Selector35/3 -> Mux/3  "<NA>"
  Bus Selector35/4 -> Mux/4  "<CB204>"
  Bus Selector35/2 -> Mux/2  "<NA>"
  Bus Selector35/16 -> Mux/16  "<CB216>"
  Bus Selector35/15 -> Mux/15  "<NA>"
  Bus Selector35/6 -> Mux/6  "<CB206>"
  Bus Selector35/8 -> Mux/8  "<CB208>"
  Bus Selector35/5 -> Mux/5  "<NA>"
  Bus Selector35/10 -> Mux/10  "<NA>"
  Bus Selector35/7 -> Mux/7  "<NA>"
  Bus Selector35/9 -> Mux/9  "<NA>"
  Bus Selector35/19 -> Mux/19  "<CB219>"
  Bus Selector35/13 -> Mux/13  "<CB213>"
  Bus Selector35/11 -> Mux/11  "<NA>"
  Bus Selector35/18 -> Mux/18  "<CB218>"
  Bus Selector35/1 -> Mux/1  "<NA>"

== system UrbanCHIL/SS_F3_RELAY_HOUSING/Subsystem ==
  bus : Inport
  Bus Selector1 : BusSelector  OutputSignals=F4.CB401,F4.CB402,F4.CB403,NA,F4.CB405,F4.CB406  OutputAsBus=on
  Bus Selector35 : BusSelector  OutputSignals=NA,NA,NA,NA,NA,NA,F3.CB307,F3.CB308,F3.CB309,F3.CB310,PCC.CB300
  Bus to Vector1 : BusToVector
  Mux : Mux  Inputs=12
  vect : Outport
  wires:
  Mux/1 -> vect/1
  Bus Selector35/9 -> Mux/9  "<CB309>"
  Bus Selector35/8 -> Mux/8  "<CB308>"
  Bus Selector35/2 -> Mux/2  "<NA>"
  Bus Selector35/5 -> Mux/5  "<NA>"
  Bus Selector35/6 -> Mux/6  "<NA>"
  Bus Selector35/10 -> Mux/10  "<CB310>"
  Bus Selector35/7 -> Mux/7  "<CB307>"
  Bus Selector35/4 -> Mux/4  "<NA>"
  Bus Selector35/11 -> Mux/11  "<CB300>"
  Bus Selector35/3 -> Mux/3  "<NA>"
  Bus Selector35/1 -> Mux/1  "<NA>"
  bus/1 -> Bus Selector1/1, Bus Selector35/1
  Bus Selector1/1 -> Bus to Vector1/1
  Bus to Vector1/1 -> Mux/12

== system UrbanCHIL/SS_Feeder2/ESS1 ==
  modbus_in : Inport
  console : Inport  Port=2
  testseq : Inport  Port=3
  Bus Creator4 : BusCreator  Inputs=3
  Bus Selector : BusSelector  OutputSignals=cb_ctrl
  Bus Selector1 : BusSelector  OutputSignals=ModbusEnable
  Bus Selector2 : BusSelector  OutputSignals=fault
  Bus Selector20 : BusSelector  OutputSignals=relay_ctrl
  Bus Selector21 : BusSelector  OutputSignals=ModbusFromSC.Ctrl,ModbusFromSC.PCmd,ModbusFromSC.QCmd,ModbusFromSC.VoltCmd,ModbusFromSC.FreqCmd,ModbusFromSC.signal6,ModbusFromSC.signal7,ModbusFromSC.signal8  OutputAsBus=on
  Bus Selector3 : BusSelector  OutputSignals=ess1
  Bus Selector4 : BusSelector  OutputSignals=Tuning
  Bus to Vector : BusToVector
  CB_ESS : breaker_lib/Breaker  Ts=Ts  mech_delay=cb_mech_delay
  Constant : Constant  Value=0
  ESS : BESS_lib/NREL_BESS  InvType=ESS Inverter  Sn=3000  Vn=480  b_Vdc_nom=1000  b_kWh=600  b_esr=0.005  r_I_max=3  Tc=Ts  MbusPrecInc=off  ExtTuningEna=on
  Generic_Relay : relay_modbus_lib/Generic_Relay_v2_1  Ts=Ts  relay_settings=[DER_REL(CBID.ESS1,:)]
  Switch : Switch  Criteria=u2 > Threshold  Threshold=0.5
  A : PMIOPort  Port=1  Side=Right
  B : PMIOPort  Port=2  Side=Right
  C : PMIOPort  Port=3  Side=Right
  modbus_out : Outport
  meas : Outport  Port=2
  wires:
  Bus Creator4/1 -> ESS/5
  Generic_Relay/2 -> Bus Creator4/2  "relay_meas"
  ESS/2 -> meas/1  "PV_meas"
  Generic_Relay/1 -> Bus Creator4/1  "relay_out"
  Bus Selector20/1 -> Generic_Relay/2  "<relay_ctrl>"
  console/1 -> Bus Selector4/1, Bus Selector1/1, Bus Selector21/1
  Bus Selector1/1 -> Switch/2  "<ModbusEnable>"
  ESS/1 -> modbus_out/1
  modbus_in/1 -> Switch/1
  Bus Selector21/1 -> Bus to Vector/1
  Switch/1 -> ESS/1
  CB_ESS/1 -> Generic_Relay/1, Bus Creator4/3  "cb_meas"
  ESS/3 -> Bus Selector20/1, Bus Selector/1
  Bus to Vector/1 -> Switch/3
  Constant/1 -> ESS/3
  testseq/1 -> Bus Selector2/1
  Bus Selector2/1 -> Bus Selector3/1  "<fault>"
  Bus Selector3/1 -> ESS/4  "<ess1>"
  Bus Selector/1 -> CB_ESS/1  "<cb_ctrl>"
  Bus Selector4/1 -> ESS/2  "<Tuning>"
  connections:
  CB_ESS/RConn2 -- B/RConn1
  ESS/RConn2 -- CB_ESS/LConn2
  ESS/RConn3 -- CB_ESS/LConn3
  ESS/RConn1 -- CB_ESS/LConn1
  A/RConn1 -- CB_ESS/RConn1
  CB_ESS/RConn3 -- C/RConn1

== system UrbanCHIL/SS_Feeder2/PV2 ==
  modbus_in : Inport
  testseq : Inport  Port=2
  console : Inport  Port=3
  Bus Creator4 : BusCreator  Inputs=3
  Bus Selector : BusSelector  OutputSignals=cb_ctrl
  Bus Selector1 : BusSelector  OutputSignals=ModbusEnable
  Bus Selector2 : BusSelector  OutputSignals=ModbusFromSC.Ctrl,ModbusFromSC.PCmd,ModbusFromSC.QCmd,ModbusFromSC.VoltCmd,ModbusFromSC.FreqCmd,ModbusFromSC.signal6,ModbusFromSC.signal7,ModbusFromSC.signal8  OutputAsBus=on
  Bus Selector20 : BusSelector  OutputSignals=relay_ctrl
  Bus Selector21 : BusSelector  OutputSignals=pv.insolation1
  Bus Selector3 : BusSelector  OutputSignals=fault
  Bus Selector4 : BusSelector  OutputSignals=pv1
  Bus Selector5 : BusSelector  OutputSignals=Tuning
  Bus to Vector : BusToVector
  F4_CB_4 : breaker_lib/Breaker  Ts=Ts  mech_delay=cb_mech_delay
  Generic_Relay : relay_modbus_lib/Generic_Relay_v2_1  Ts=Ts  relay_settings=[DER_REL(CBID.PV1,:)]
  Inverter : BESS_lib/NREL_BESS  InvType=PV Inverter  Sn=5000  Vn=480  b_Vdc_nom=1000  b_kWh=1000  b_esr=0.002  r_I_max=1.2  Tc=Ts  MbusPrecInc=off  ExtTuningEna=on
  Switch : Switch  Criteria=u2 > Threshold  Threshold=0.5
  A : PMIOPort  Port=1  Side=Right
  B : PMIOPort  Port=2  Side=Right
  C : PMIOPort  Port=3  Side=Right
  modbus_out : Outport
  meas : Outport  Port=2
  wires:
  Inverter/3 -> Bus Selector20/1, Bus Selector/1
  F4_CB_4/1 -> Bus Creator4/3, Generic_Relay/1  "cb_meas"
  Switch/1 -> Inverter/1
  modbus_in/1 -> Switch/1
  Inverter/1 -> modbus_out/1
  Bus Selector20/1 -> Generic_Relay/2  "<relay_ctrl>"
  Generic_Relay/1 -> Bus Creator4/1  "relay_out"
  Inverter/2 -> meas/1  "PV_meas"
  Generic_Relay/2 -> Bus Creator4/2  "relay_meas"
  Bus Creator4/1 -> Inverter/5
  Bus Selector21/1 -> Inverter/3  "<insolation1>"
  Bus to Vector/1 -> Switch/3
  console/1 -> Bus Selector5/1, Bus Selector2/1, Bus Selector1/1
  Bus Selector1/1 -> Switch/2  "<ModbusEnable>"
  Bus Selector2/1 -> Bus to Vector/1
  testseq/1 -> Bus Selector3/1, Bus Selector21/1
  Bus Selector3/1 -> Bus Selector4/1  "<fault>"
  Bus Selector4/1 -> Inverter/4  "<pv1>"
  Bus Selector/1 -> F4_CB_4/1  "<cb_ctrl>"
  Bus Selector5/1 -> Inverter/2  "<Tuning>"
  connections:
  F4_CB_4/RConn3 -- C/RConn1
  A/RConn1 -- F4_CB_4/RConn1
  Inverter/RConn1 -- F4_CB_4/LConn1
  Inverter/RConn3 -- F4_CB_4/LConn3
  Inverter/RConn2 -- F4_CB_4/LConn2
  F4_CB_4/RConn2 -- B/RConn1
